simulink model "simulation_quad_vol"  (R2020b)
settings: Solver=VariableStepAuto  StartTime=0.0  StopTime=10  RelTol=1e-3
values from neighbouring files (symbols this model uses):
  controlleur = struct('kv',2.0,                       'k1',1.0,                       'kc',1.0,                       'kpd',8.0,                       'k_delta',15.0,                       'u_barre',u_barre,                       'M_k',M_k,                       'skew_sym_d_etoile',skew_sym_d_etoile,                       'd_etoile', d_etoile                       )    [generateContolleur.m]    (also in run_quad_vol.m = generateContolleur(drone))
  drone = struct('MASS',               0.5,                      'INERTIA',            eye(3),                     'G',                  9.81,                       'Mb',                 zeros(3,4),                 'Fb',                 zeros(3,4)                 )    [generatequad.m]    (also in run_quad_vol.m = generatequad())
  initial_state = [p_initial; v_initial; omega_initial; q_initial]    [run_quad_vol.m]
  p2 = [1000; 1000; 0]    [run_quad_vol.m]
  vitesse_cible = 5    [run_quad_vol.m]
settings Model: Creator=florian  LastModifiedBy=florian

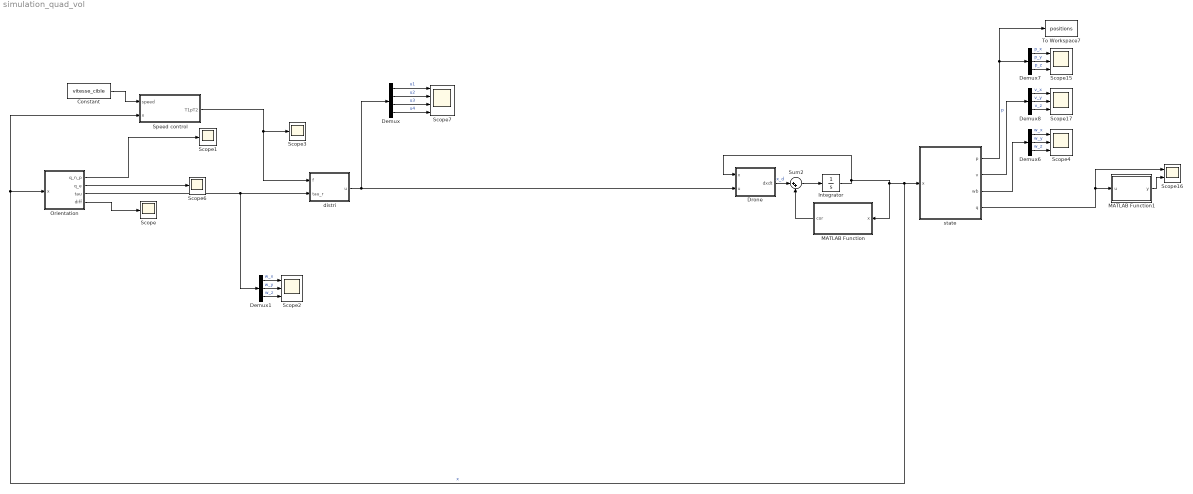
== system simulation_quad_vol ==
  Constant : Constant  Value=vitesse_cible
  Demux : Demux
  Demux{1,6..8} (4 alike) : Demux  Outputs=3
  Drone : MATLAB Function  TreatAsAtomicUnit=on
  Integrator : Integrator  InitialCondition=initial_state
  MATLAB Function : MATLAB Function  TreatAsAtomicUnit=on
  MATLAB Function1 : MATLAB Function  TreatAsAtomicUnit=on
  Orientation : MATLAB Function  TreatAsAtomicUnit=on
  Scope{,1,3,6} (4 alike) : Scope
  Scope{2,4,15,17} (4 alike) : Scope  NumInputPorts=3
  Scope16 : Scope  NumInputPorts=2
  Scope7 : Scope  NumInputPorts=4
  Speed control : MATLAB Function  TreatAsAtomicUnit=on
  Sum2 : Sum  Inputs=|++
  To Workspace7 : ToWorkspace  VariableName=positions  SampleTime=-1
  distri : MATLAB Function  TreatAsAtomicUnit=on
  state : MATLAB Function  TreatAsAtomicUnit=on
  wires:
  Demux7/2 -> Scope15/2  "p_y"
  state/1(p) -> To Workspace7/1, Demux7/1  "p"
  state/4(q) -> Scope16/1, MATLAB Function1/1(u)
  Demux8/3 -> Scope17/3  "v_z"
  Demux8/1 -> Scope17/1  "v_x"
  MATLAB Function1/1(y) -> Scope16/2
  Demux8/2 -> Scope17/2  "v_y"
  state/2(v) -> Demux8/1
  Demux7/1 -> Scope15/1  "p_x"
  Demux7/3 -> Scope15/3  "p_z"
  Drone/1(dxdt) -> Sum2/1  "x_d"
  Sum2/1 -> Integrator/1
  MATLAB Function/1(cor) -> Sum2/2
  Demux6/2 -> Scope4/2  "w_y"
  Demux6/3 -> Scope4/3  "w_z"
  state/3(wb) -> Demux6/1
  Demux6/1 -> Scope4/1  "w_x"
  distri/1(u) -> Drone/2(u), Demux/1
  Demux/4 -> Scope7/4  "u4"
  Demux/2 -> Scope7/2  "u2"
  Demux/3 -> Scope7/3  "u3"
  Demux/1 -> Scope7/1  "u1"
  Constant/1 -> Speed control/1(speed)
  Integrator/1 -> Drone/1(x), MATLAB Function/1(x), Speed control/2(x), Orientation/1(x), state/1(x)  "x"
  Orientation/4(diff) -> Scope/1
  Orientation/1(q_n_p) -> Scope1/1
  Speed control/1(T1pT2) -> Scope3/1, distri/1(f)
  Orientation/2(q_e) -> Scope6/1
  Orientation/3(tau) -> Demux1/1, distri/2(tau_r)
  Demux1/2 -> Scope2/2  "w_y"
  Demux1/3 -> Scope2/3  "w_z"
  Demux1/1 -> Scope2/1  "w_x"

== matlab function simulation_quad_vol/Drone ==
  data: x input; u input; dxdt output; drone parameter
function dxdt = drone(x, u, drone)

%% physical constants
% gravity
g = drone.G;
% vehicle mass
m = drone.MASS;
% vehicle inertia matrix
J = drone.INERTIA; % [3x3 real symmetric] in body axis

%% state demultiplexing
% p = x(1:3);
v = x(4:6);
wb = x(7:9);
q  = x(10:13);

Rq = q2dcm(q);

% position
dpdt = v;

% kinematics
dvdt =  -[0;0;g] + (1/m)*Rq*drone.Fb*u; 

%% angular velocity derivative
% kinematics
dwdt = -J\cross(wb, J*wb) + J\(drone.Mb*u);

%% quaternion derivative
eta = q(1);
eps = q(2:4);

dqdt = (1/2)*[-eps'; eta*eye(3) + skew_sym(eps)]*wb;

%% derivative multiplexing
dxdt = [dpdt; dvdt; dwdt; dqdt] ;

== matlab function simulation_quad_vol/Speed control ==
  data: speed input; x input; T1pT2 output; controlleur parameter; drone parameter
function T1pT2 = speed_control(speed, x, controlleur, drone)
%#codegen 

% p = x(1:3);
v = x(4:6);
%q  = x(7:10);
% w = x(11:13);


T1pT2 =  controlleur.kv * (speed - v(1));

== matlab function simulation_quad_vol/distri ==
  data: f input; u output; tau_r input; controlleur parameter
function u = dist(f,tau_r, controlleur)
%#codegen
u = controlleur.M_k * tau_r + controlleur.u_barre * f;

== matlab function simulation_quad_vol/Orientation ==
  data: q_n_p output; q_e output; x input; tau output; p2 parameter; controlleur parameter; drone parameter; diff output
function [q_n_p, q_e, tau, diff]= orientation(x, p2, controlleur, drone)
%#codegen
p = x(1:3);
% v = x(4:6);
q  = x(7:10);


u_p = (p2-p)/norm(p2-p);

khi_p = atan2(u_p(1), u_p(2));
gamma_p = -atan2(u_p(3), sqrt(u_p(1)^2 + u_p(2)^2));

q_p_khi = [cos(khi_p/2); 0; 0; sin(khi_p/2)];
q_p_gamma = [cos(gamma_p/2); 0; sin(gamma_p/2); 0];

q_n_p = quadprod(q_p_khi, q_p_gamma);
q_e = quadprod(quadconj(q_n_p), q);

tau = -controlleur.kc*q_e(1)*q_e(2:4);

diff = q-q_e;

== matlab function simulation_quad_vol/MATLAB Function1 ==
  data: u input; y output
function y = fcn(u)
%#codegen

y = norm(u);

== matlab function simulation_quad_vol/state ==
  data: x input; p output; v output; wb output; q output
function [p, v, wb, q]= demux(x)
%#codegen

p = x(1:3);
v = x(4:6);
wb = x(7:9);
q  = x(10:13);

== matlab function simulation_quad_vol/MATLAB Function ==
  data: x input; cor output
function cor  = fcn(x)
%#codegen
q  = x(10:13);
n = norm(q);
mismatch = 1-n;
cor = [0;0;0; 0;0;0; 0;0;0; mismatch*q];
